simulink library "IEEE9BusTestSystem"  (R2018a)
settings: Solver=VariableStepAuto  StartTime=0.0  StopTime=10.0  RelTol=1e-3
values from neighbouring files (symbols this model uses):
  C_4 = 0.1670*C_b    (= 1.00487241952e-06)    [VSM.m]    (also in dVOC.m; droop.m; droop_with_current_limitation.m; matching.m)
  C_6 = 0.2835*C_b    (= 1.70587623314e-06)    [VSM.m]    (also in dVOC.m; droop.m; droop_with_current_limitation.m; matching.m)
  C_8 = 0.2275*C_b    (= 1.36891302659e-06)    [VSM.m]    (also in dVOC.m; droop.m; droop_with_current_limitation.m; matching.m)
  L_45 = L_lines(2)    [VSM.m]    (also in dVOC.m; droop.m; droop_with_current_limitation.m; matching.m)
  L_56 = L_lines(3)    [VSM.m]    (also in dVOC.m; droop.m; droop_with_current_limitation.m; matching.m)
  L_67 = L_lines(5)    [VSM.m]    (also in dVOC.m; droop.m; droop_with_current_limitation.m; matching.m)
  L_78 = L_lines(6)    [VSM.m]    (also in dVOC.m; droop.m; droop_with_current_limitation.m; matching.m)
  L_89 = L_lines(8)    [VSM.m]    (also in dVOC.m; droop.m; droop_with_current_limitation.m; matching.m)
  L_94 = L_lines(9)    [VSM.m]    (also in dVOC.m; droop.m; droop_with_current_limitation.m; matching.m)
  R_45 = R_lines(2)    [VSM.m]    (also in dVOC.m; droop.m; droop_with_current_limitation.m; matching.m)
  R_56 = R_lines(3)    [VSM.m]    (also in dVOC.m; droop.m; droop_with_current_limitation.m; matching.m)
  R_67 = R_lines(5)    [VSM.m]    (also in dVOC.m; droop.m; droop_with_current_limitation.m; matching.m)
  R_78 = R_lines(6)    [VSM.m]    (also in dVOC.m; droop.m; droop_with_current_limitation.m; matching.m)
  R_89 = R_lines(8)    [VSM.m]    (also in dVOC.m; droop.m; droop_with_current_limitation.m; matching.m)
  R_94 = R_lines(9)    [VSM.m]    (also in dVOC.m; droop.m; droop_with_current_limitation.m; matching.m)
  V2_rms = 13800    [VSM.m]    (also in dVOC.m; droop.m; droop_with_current_limitation.m; matching.m)
undefined symbols (not defined in the file or in its folder): D1, Delta
libraries: powerlib x27
settings Model: Creator=TayyebiA  LastModifiedBy=TayyebiA

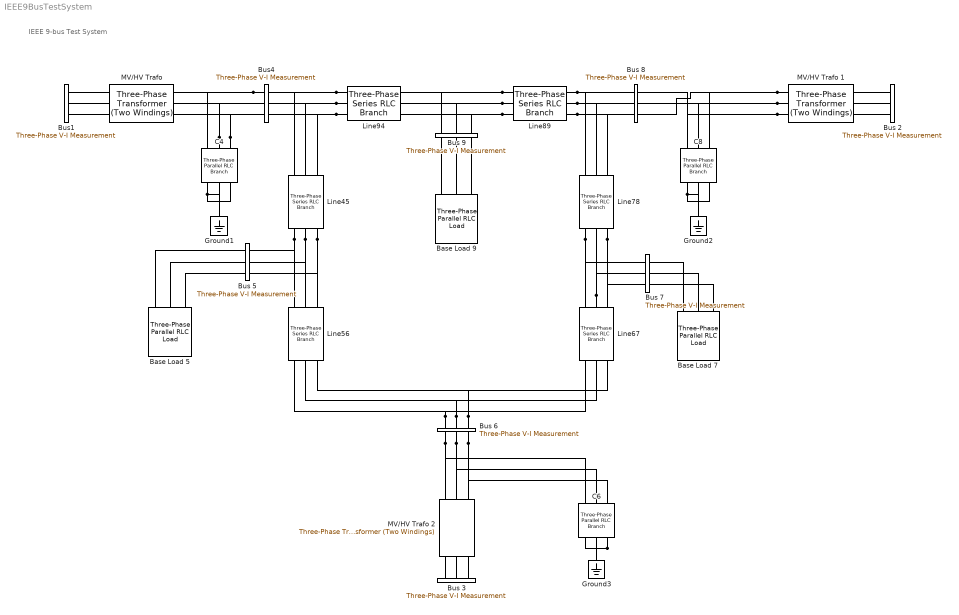
== system IEEE9BusTestSystem ==
  note: IEEE 9-bus Test System
  Base Load 5 : powerlib/Elements/Three-Phase Parallel RLC Load  LConnTagsString=A|B|C  Configuration=Y (grounded)  NominalVoltage=230e3  Vabc=[1e3 1e3 1e3]  Vabcp=[1e3 1e3 1e3]  NominalFrequency=50  UnbalancedPower=off  ActivePower=pl  InductivePower=0  CapacitivePower=0  Pabc=[10e3 9e3 11e3]  QLabc=[100 90 110]  QCabc=[100 90 110]  Pabcp=[10e3 9e3 11e3]  QLabcp=[100 90 110]  QCabcp=[100 90 110]  Measurements=None  LoadType=constant Z
  Base Load 7 : powerlib/Elements/Three-Phase Parallel RLC Load  LConnTagsString=A|B|C  Configuration=Y (grounded)  NominalVoltage=230e3  Vabc=[1e3 1e3 1e3]  Vabcp=[1e3 1e3 1e3]  NominalFrequency=50  UnbalancedPower=off  ActivePower=pl  InductivePower=0  CapacitivePower=0  Pabc=[10e3 9e3 11e3]  QLabc=[100 90 110]  QCabc=[100 90 110]  Pabcp=[10e3 9e3 11e3]  QLabcp=[100 90 110]  QCabcp=[100 90 110]  Measurements=None  LoadType=constant Z
  "Base Load 9 " : powerlib/Elements/Three-Phase Parallel RLC Load  LConnTagsString=A|B|C  Configuration=Y (grounded)  NominalVoltage=230e3  Vabc=[1e3 1e3 1e3]  Vabcp=[1e3 1e3 1e3]  NominalFrequency=50  UnbalancedPower=off  ActivePower=pl  InductivePower=0  CapacitivePower=0  Pabc=[10e3 9e3 11e3]  QLabc=[100 90 110]  QCabc=[100 90 110]  Pabcp=[10e3 9e3 11e3]  QLabcp=[100 90 110]  QCabcp=[100 90 110]  Measurements=None  LoadType=constant Z
  Bus 2 : powerlib/Measurements/Three-Phase V-I Measurement  VoltageMeasurement=no  SetLabelV=on  LabelV=Vabc_8  Vpu=on  VpuLL=off  CurrentMeasurement=no  SetLabelI=on  LabelI=Iabc_8  Ipu=on  Pbase=S_b  Vbase=V_b  OutputType=Complex  PhasorSimulation=off  PSBequivalent=0
  Bus 3 : powerlib/Measurements/Three-Phase V-I Measurement  VoltageMeasurement=no  SetLabelV=off  LabelV=Vabc_6  Vpu=off  VpuLL=off  CurrentMeasurement=no  SetLabelI=off  LabelI=Iabc_6  Ipu=off  Pbase=S_b  Vbase=V_b  OutputType=Complex  PhasorSimulation=off  PSBequivalent=0
  Bus 5 : powerlib/Measurements/Three-Phase V-I Measurement  VoltageMeasurement=no  SetLabelV=on  LabelV=Vabc_5  Vpu=on  VpuLL=off  CurrentMeasurement=no  SetLabelI=on  LabelI=Iabc_5  Ipu=on  Pbase=S_b  Vbase=V_b  OutputType=Complex  PhasorSimulation=off  PSBequivalent=0
  Bus 6 : powerlib/Measurements/Three-Phase V-I Measurement  VoltageMeasurement=no  SetLabelV=off  LabelV=Vabc_6  Vpu=off  VpuLL=off  CurrentMeasurement=no  SetLabelI=off  LabelI=Iabc_6  Ipu=off  Pbase=S_b  Vbase=V_b  OutputType=Complex  PhasorSimulation=off  PSBequivalent=0
  Bus 7 : powerlib/Measurements/Three-Phase V-I Measurement  VoltageMeasurement=no  SetLabelV=on  LabelV=Vabc_5  Vpu=on  VpuLL=off  CurrentMeasurement=no  SetLabelI=on  LabelI=Iabc_5  Ipu=on  Pbase=S_b  Vbase=V_b  OutputType=Complex  PhasorSimulation=off  PSBequivalent=0
  Bus 8 : powerlib/Measurements/Three-Phase V-I Measurement  VoltageMeasurement=no  SetLabelV=on  LabelV=Vabc_8  Vpu=on  VpuLL=off  CurrentMeasurement=no  SetLabelI=on  LabelI=Iabc_8  Ipu=on  Pbase=S_b  Vbase=V_b  OutputType=Complex  PhasorSimulation=off  PSBequivalent=0
  Bus 9 : powerlib/Measurements/Three-Phase V-I Measurement  VoltageMeasurement=no  SetLabelV=on  LabelV=Vabc_9  Vpu=on  VpuLL=off  CurrentMeasurement=no  SetLabelI=on  LabelI=Iabc_9  Ipu=on  Pbase=S_b  Vbase=V_b  OutputType=Complex  PhasorSimulation=off  PSBequivalent=0
  Bus1 : powerlib/Measurements/Three-Phase V-I Measurement  VoltageMeasurement=no  SetLabelV=on  LabelV=Vabc_1  Vpu=on  VpuLL=off  CurrentMeasurement=no  SetLabelI=on  LabelI=Iabc_1  Ipu=on  Pbase=S_b  Vbase=V_b  OutputType=Complex  PhasorSimulation=off  PSBequivalent=0
  Bus4 : powerlib/Measurements/Three-Phase V-I Measurement  VoltageMeasurement=no  SetLabelV=on  LabelV=Vabc_4  Vpu=on  VpuLL=off  CurrentMeasurement=no  SetLabelI=on  LabelI=Iabc_4  Ipu=on  Pbase=S_b  Vbase=V_b  OutputType=Complex  PhasorSimulation=off  PSBequivalent=0
  C4 : powerlib/Elements/Three-Phase Parallel RLC Branch  LConnTagsString=A|B|C  RConnTagsString=A|B|C  BranchType=C  Resistance=1  Inductance=1e-3  Capacitance=C_4  Measurements=None
      settings: SourceProductName=Simscape Power Systems  SourceProductBaseCode=PS
  C6 : powerlib/Elements/Three-Phase Parallel RLC Branch  LConnTagsString=A|B|C  RConnTagsString=A|B|C  BranchType=C  Resistance=1  Inductance=1e-3  Capacitance=C_6  Measurements=None
      settings: SourceProductName=Simscape Power Systems  SourceProductBaseCode=PS
  C8 : powerlib/Elements/Three-Phase Parallel RLC Branch  LConnTagsString=A|B|C  RConnTagsString=A|B|C  BranchType=C  Resistance=1  Inductance=1e-3  Capacitance=C_8  Measurements=None
      settings: SourceProductName=Simscape Power Systems  SourceProductBaseCode=PS
  Ground1 : powerlib/Elements/Ground  LConnTagsString=a
  Ground2 : powerlib/Elements/Ground  LConnTagsString=a
  Ground3 : powerlib/Elements/Ground  LConnTagsString=a
  Line45 : powerlib/Elements/Three-Phase Series RLC Branch  LConnTagsString=A|B|C  RConnTagsString=A|B|C  BranchType=RL  Resistance=R_45  Inductance=L_45  Capacitance=0  Measurements=None
  Line56 : powerlib/Elements/Three-Phase Series RLC Branch  LConnTagsString=A|B|C  RConnTagsString=A|B|C  BranchType=RL  Resistance=R_56  Inductance=L_56  Capacitance=0  Measurements=None
  Line67 : powerlib/Elements/Three-Phase Series RLC Branch  LConnTagsString=A|B|C  RConnTagsString=A|B|C  BranchType=RL  Resistance=R_67  Inductance=L_67  Capacitance=0  Measurements=None
  Line78 : powerlib/Elements/Three-Phase Series RLC Branch  LConnTagsString=A|B|C  RConnTagsString=A|B|C  BranchType=RL  Resistance=R_78  Inductance=L_78  Capacitance=0  Measurements=None
  Line89 : powerlib/Elements/Three-Phase Series RLC Branch  LConnTagsString=A|B|C  RConnTagsString=A|B|C  BranchType=RL  Resistance=R_89  Inductance=L_89  Capacitance=0  Measurements=None
  Line94 : powerlib/Elements/Three-Phase Series RLC Branch  LConnTagsString=A|B|C  RConnTagsString=A|B|C  BranchType=RL  Resistance=R_94  Inductance=L_94  Capacitance=0  Measurements=None
  "MV/HV Trafo " : powerlib/Elements/Three-Phase Transformer (Two Windings)  Winding1Connection=Delta (D1)  Winding2Connection=Yg  CoreType=Three single-phase transformers  SetSaturation=off  Hysteresis=off  DataFile='hysteresis'  SetInitialFlux=off  Measurements=None  UNITS=pu  NominalPower=[ 210e6 50 ]  Winding1="[V2_rms 0.0027  0.08]"  Winding2=[230e3 0.0027 0.08]  Rm=500  Lm=500  L0=0.5  Saturation="[ 0,0  ;  0.005,1.2  ;  1.0,1.4 ]"  InitialFluxes=[ 0.8 , -0.8 , 0.7 ]  MoreParameters=off  BreakLoop=off  DataType=off  TransfoNumber=0
  "MV/HV Trafo 1 " : powerlib/Elements/Three-Phase Transformer (Two Windings)  Winding1Connection=Yg  Winding2Connection=Yg  CoreType=Three single-phase transformers  SetSaturation=off  Hysteresis=off  DataFile='hysteresis'  SetInitialFlux=off  Measurements=None  UNITS=pu  NominalPower=[ 210e6 50 ]  Winding1=[V2_rms 0.0027 0.08]  Winding2=[ 230e3 0.0027 0.08]  Rm=500  Lm=500  L0=0.5  Saturation="[ 0,0  ;  0.005,1.2  ;  1.0,1.4 ]"  InitialFluxes=[ 0.8 , -0.8 , 0.7 ]  MoreParameters=off  BreakLoop=off  DataType=off  TransfoNumber=0
  "MV/HV Trafo 2 " : powerlib/Elements/Three-Phase Transformer (Two Windings)  Winding1Connection=Yg  Winding2Connection=Yg  CoreType=Three single-phase transformers  SetSaturation=off  Hysteresis=off  DataFile='hysteresis'  SetInitialFlux=off  Measurements=None  UNITS=pu  NominalPower=[ 210e6 50 ]  Winding1=[V2_rms 0.0027 0.08]  Winding2=[230e3 0.0027 0.08]  Rm=500  Lm=500  L0=0.5  Saturation="[ 0,0  ;  0.005,1.2  ;  1.0,1.4 ]"  InitialFluxes=[ 0.8 , -0.8 , 0.7 ]  MoreParameters=off  BreakLoop=off  DataType=off  TransfoNumber=0
  connections:
  C8/RConn1 -- C8/RConn2 -- C8/RConn3 -- Ground2/LConn1
  "MV/HV Trafo 1 "/RConn3 -- Bus 8/LConn3 -- C8/LConn3
  Line78/RConn1 -- Line67/LConn1 -- Bus 7/RConn1
  Bus 6/LConn3 -- Line67/RConn3 -- Line56/RConn3
  Line89/LConn3 -- Line94/RConn3 -- Bus 9/RConn1
  C4/LConn3 -- Bus4/RConn3 -- "MV/HV Trafo "/RConn3
  Bus 6/LConn1 -- Line67/RConn1 -- Line56/RConn1
  Line67/LConn2 -- Line78/RConn2 -- Bus 7/RConn2
  Line89/LConn1 -- Line94/RConn1 -- Bus 9/RConn3
  "MV/HV Trafo 1 "/RConn1 -- Bus 8/LConn1 -- C8/LConn1
  Line45/RConn2 -- Line56/LConn2 -- Bus 5/LConn2
  Bus4/RConn1 -- "MV/HV Trafo "/RConn1 -- C4/LConn1
  C4/RConn1 -- Ground1/LConn1 -- C4/RConn2 -- C4/RConn3
  Line89/RConn3 -- Bus 8/RConn3 -- Line78/LConn3
  Line94/LConn3 -- Bus4/LConn3 -- Line45/LConn3
  Bus 6/RConn2 -- C6/LConn2 -- "MV/HV Trafo 2 "/RConn2
  Line89/RConn2 -- Bus 8/RConn2 -- Line78/LConn2
  Line89/LConn2 -- Bus 9/RConn2 -- Line94/RConn2
  Bus 6/RConn3 -- "MV/HV Trafo 2 "/RConn3 -- C6/LConn3
  Line45/RConn3 -- Line56/LConn3 -- Bus 5/LConn3
  "MV/HV Trafo 1 "/RConn2 -- Bus 8/LConn2 -- C8/LConn2
  Bus 6/LConn2 -- Line67/RConn2 -- Line56/RConn2
  Line94/LConn1 -- Bus4/LConn1 -- Line45/LConn1
  Line78/RConn3 -- Line67/LConn3 -- Bus 7/RConn3
  Line94/LConn2 -- Bus4/LConn2 -- Line45/LConn2
  C6/RConn3 -- C6/RConn2 -- C6/RConn1 -- Ground3/LConn1
  Line89/RConn1 -- Bus 8/RConn1 -- Line78/LConn1
  Bus 6/RConn1 -- C6/LConn1 -- "MV/HV Trafo 2 "/RConn1
  C4/LConn2 -- Bus4/RConn2 -- "MV/HV Trafo "/RConn2
  Line45/RConn1 -- Line56/LConn1 -- Bus 5/LConn1
  "Base Load 9 "/LConn2 -- Bus 9/LConn2
  Bus1/LConn3 -- "MV/HV Trafo "/LConn3
  Bus 2/RConn3 -- "MV/HV Trafo 1 "/LConn1
  Bus 3/LConn1 -- "MV/HV Trafo 2 "/LConn1
  Bus 3/LConn3 -- "MV/HV Trafo 2 "/LConn3
  Bus1/LConn2 -- "MV/HV Trafo "/LConn2
  Base Load 5/LConn2 -- Bus 5/RConn2
  Base Load 5/LConn1 -- Bus 5/RConn1
  Bus 2/RConn1 -- "MV/HV Trafo 1 "/LConn3
  "Base Load 9 "/LConn1 -- Bus 9/LConn3
  Bus 7/LConn2 -- Base Load 7/LConn2
  "Base Load 9 "/LConn3 -- Bus 9/LConn1
  Bus 2/RConn2 -- "MV/HV Trafo 1 "/LConn2
  Bus 7/LConn1 -- Base Load 7/LConn1
  Bus 3/LConn2 -- "MV/HV Trafo 2 "/LConn2
  Bus1/LConn1 -- "MV/HV Trafo "/LConn1
  Base Load 5/LConn3 -- Bus 5/RConn3
  Bus 7/LConn3 -- Base Load 7/LConn3
